simulink model "TADPOLE_Closed_Loop_CTRL2"  (R2024b)
settings: Solver=ode45  StartTime=0.0  StopTime=19  RelTol=1e-3
InitFcn:
  | clear mex;
values from neighbouring files (symbols this model uses):
  timeDelta = 1/5000    (= 0.0002)    [TADPOLEControl.m]
undefined symbols (not defined in the file or in its folder): DiscIntNeverNeededParam
settings Model: PacingRate=2  Creator=pplat  LastModifiedBy=pplat
settings DebuggingCC: AlgebraicLoopMsg=none

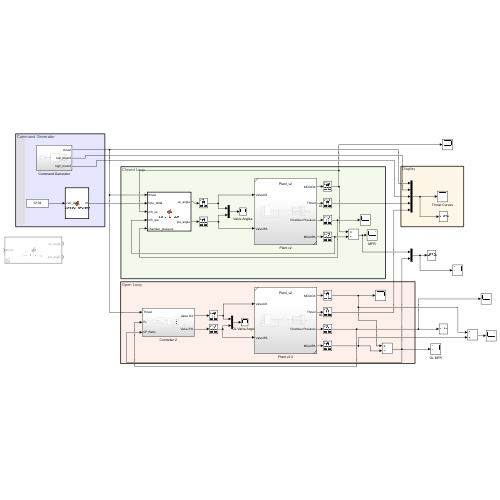
[thumbnail: Simulink's stored preview of the top-level diagram]
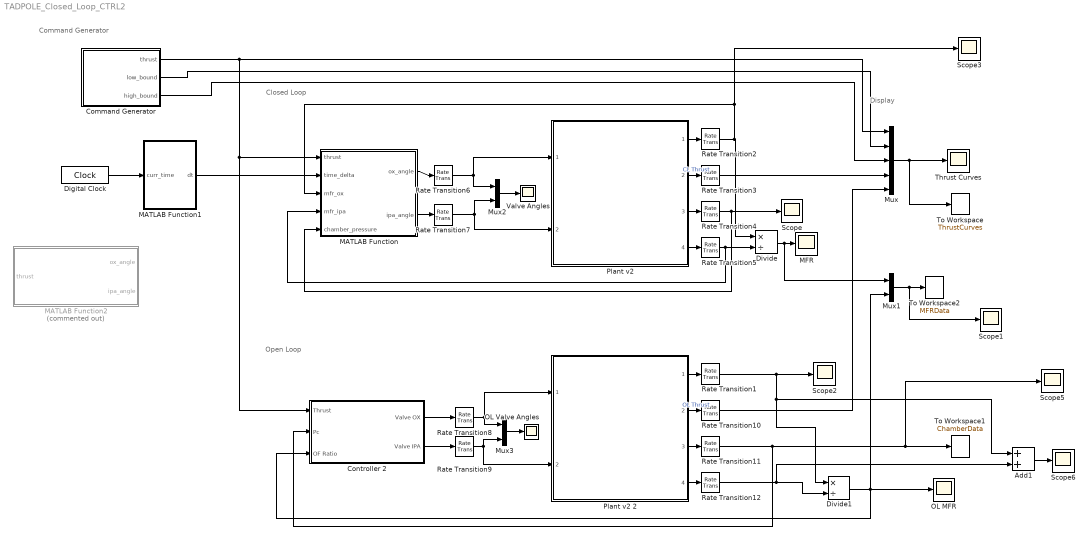
== system TADPOLE_Closed_Loop_CTRL2 ==
  note: Display
  note: Open Loop
  note: Closed Loop
  note: Command Generator
  Add1 : Sum
  Command Generator : Subsystem
  Controller 2 : Subsystem
  Digital Clock : DigitalClock  SampleTime=timeDelta
  Divide : Product  Inputs=*/
  Divide1 : Product  Inputs=*/
  MATLAB Function : MATLAB Function  TreatAsAtomicUnit=on
  MATLAB Function1 : MATLAB Function  TreatAsAtomicUnit=on
  MATLAB Function2 : MATLAB Function  Commented=on  TreatAsAtomicUnit=on
  MFR : Scope
  Mux : Mux  Inputs=5
  Mux1 : Mux  Inputs=2
  Mux2 : Mux  Inputs=2
  Mux3 : Mux  Inputs=2
  OL MFR : Scope
  OL Valve Angles : Scope
  Plant v2 : Subsystem  ReferencedSubsystem=Plant_v2
  Plant v2 2 : Subsystem  ReferencedSubsystem=Plant_v2
  Rate Transition{1..5,10..12} (8 alike) : RateTransition  OutPortSampleTime=timeDeltaOUT
  Rate Transition{6..9} (4 alike) : RateTransition  OutPortSampleTime=timeDeltaCMD
  Scope{,1..3,5..6} (6 alike) : Scope
  Thrust Curves : Scope
  To Workspace : ToWorkspace  VariableName=ThrustCurves  SaveFormat=Timeseries  SampleTime=-1
  To Workspace1 : ToWorkspace  VariableName=ChamberData  SaveFormat=Timeseries  SampleTime=-1
  To Workspace2 : ToWorkspace  VariableName=MFRData  SaveFormat=Timeseries  SampleTime=-1
  Valve Angles : Scope
  wires:
  Mux/1 -> To Workspace/1, Thrust Curves/1
  Plant v2/4 -> Rate Transition5/1
  MATLAB Function/2(ipa_angle) -> Rate Transition7/1
  MATLAB Function/1(ox_angle) -> Rate Transition6/1
  Mux2/1 -> Valve Angles/1
  Divide/1 -> Mux1/1, MFR/1
  Command Generator/1(thrust) -> Mux/1, Controller 2/1(Thrust), MATLAB Function/1(thrust)
  Plant v2/2 -> Rate Transition3/1  "CL Thrust"
  Command Generator/2(low_bound) -> Mux/2
  Command Generator/3(high_bound) -> Mux/3
  MATLAB Function1/1(dt) -> MATLAB Function/2(time_delta)
  Mux3/1 -> OL Valve Angles/1
  Divide1/1 -> Mux1/2, Controller 2/3(OF Ratio), OL MFR/1
  Controller 2/1(Valve OX) -> Rate Transition8/1
  Controller 2/2(Valve IPA) -> Rate Transition9/1
  Digital Clock/1 -> MATLAB Function1/1(curr_time)
  Plant v2 2/1 -> Rate Transition1/1
  Plant v2 2/4 -> Rate Transition12/1
  Mux1/1 -> Scope1/1, To Workspace2/1
  Plant v2/3 -> Rate Transition4/1
  Plant v2 2/3 -> Rate Transition11/1
  Plant v2/1 -> Rate Transition2/1
  Add1/1 -> Scope6/1
  Rate Transition2/1 -> Divide/1, Scope3/1, MATLAB Function/3(mfr_ox)
  Rate Transition3/1 -> Mux/4
  Rate Transition4/1 -> MATLAB Function/5(chamber_pressure), Scope/1
  Rate Transition5/1 -> Divide/2, MATLAB Function/4(mfr_ipa)
  Rate Transition6/1 -> Plant v2/1, Mux2/1
  Rate Transition7/1 -> Plant v2/2, Mux2/2
  Rate Transition8/1 -> Plant v2 2/1, Mux3/1
  Rate Transition9/1 -> Plant v2 2/2, Mux3/2
  Rate Transition1/1 -> Scope2/1, Add1/1, Divide1/1
  Rate Transition10/1 -> Mux/5
  Plant v2 2/2 -> Rate Transition10/1  "OL Thrust"
  Rate Transition11/1 -> Controller 2/2(Pc), Scope5/1, To Workspace1/1
  Rate Transition12/1 -> Add1/2, Divide1/2

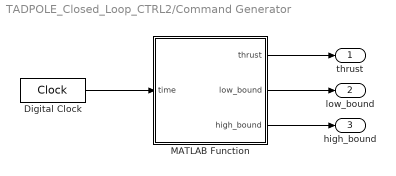
== system TADPOLE_Closed_Loop_CTRL2/Command Generator ==
  Digital Clock : DigitalClock  SampleTime=timeDelta
  MATLAB Function : MATLAB Function  TreatAsAtomicUnit=on
  thrust : Outport
  low_bound : Outport  Port=2
  high_bound : Outport  Port=3
  wires:
  MATLAB Function/1(thrust) -> thrust/1
  Digital Clock/1 -> MATLAB Function/1(time)
  MATLAB Function/2(low_bound) -> low_bound/1
  MATLAB Function/3(high_bound) -> high_bound/1

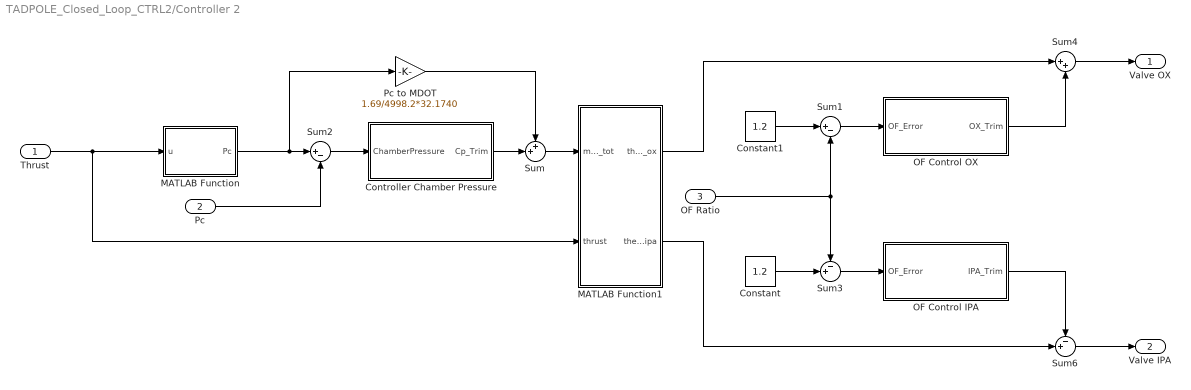
== system TADPOLE_Closed_Loop_CTRL2/Controller 2 ==
  Thrust : Inport
  Pc : Inport  Port=2
  OF Ratio : Inport  Port=3
  Constant : Constant  Value=1.2
  Constant1 : Constant  Value=1.2
  Controller Chamber Pressure : Subsystem
      settings: PortSchema="{\"entries\":[{\"content\":{\"sides\":[{\"content\":{\"connectorIds\":[\"Out1\"]},\"type\":\"ConnectorPlacement.EquallySpacedRectSide\",\"uuid\":\"33f68c87-1ae2-45d4-8ad9-4cf3c5bc8584\"},{\"content\":{\"connectorIds\":[\"In1\"],\"side\":\"RIGHT\"},\"type\":\"ConnectorPlacement.EquallySpacedRectSide\",\"uuid\":\"17976ab6-0faa-4d7d-91ba-f8a21a62dc32\"},{\"content\":{\"side\":\"TOP\"},\"type\":\"ConnectorPlacement.EquallySpacedRectSide\",\"uuid\":\"89a256ba-7dd2-41f4-a68b-27cc674e20da\"},{\"content\":{\"side\":\"BOTTOM\"},\"type\":\"ConnectorPlacement.EquallySpacedRectSide\",\"uuid\":\"73e60893-e40b-4ea1-8c2d-1d944b0843d3\"}]},\"type\":\"ConnectorPlacement.EquallySpacedConnector\",\"uuid\":\"c17bed4f-f3ae-43fd-abcb-ba9ac56db614\"}],\"packageUris\":[\"http://schema.mathworks.com/mf0/Connector/R2020b\"],\"version\":\"1.0\"}"
  MATLAB Function : MATLAB Function  TreatAsAtomicUnit=on
  MATLAB Function1 : MATLAB Function  TreatAsAtomicUnit=on
  OF Control IPA : Subsystem
      settings: PortSchema="{\"entries\":[{\"content\":{\"sides\":[{\"content\":{\"connectorIds\":[\"Out1\"]},\"type\":\"ConnectorPlacement.EquallySpacedRectSide\",\"uuid\":\"33f68c87-1ae2-45d4-8ad9-4cf3c5bc8584\"},{\"content\":{\"connectorIds\":[\"In1\"],\"side\":\"RIGHT\"},\"type\":\"ConnectorPlacement.EquallySpacedRectSide\",\"uuid\":\"17976ab6-0faa-4d7d-91ba-f8a21a62dc32\"},{\"content\":{\"side\":\"TOP\"},\"type\":\"ConnectorPlacement.EquallySpacedRectSide\",\"uuid\":\"89a256ba-7dd2-41f4-a68b-27cc674e20da\"},{\"content\":{\"side\":\"BOTTOM\"},\"type\":\"ConnectorPlacement.EquallySpacedRectSide\",\"uuid\":\"73e60893-e40b-4ea1-8c2d-1d944b0843d3\"}]},\"type\":\"ConnectorPlacement.EquallySpacedConnector\",\"uuid\":\"c17bed4f-f3ae-43fd-abcb-ba9ac56db614\"}],\"packageUris\":[\"http://schema.mathworks.com/mf0/Connector/R2020b\"],\"version\":\"1.0\"}"
  OF Control OX : Subsystem
      settings: PortSchema="{\"entries\":[{\"content\":{\"sides\":[{\"content\":{\"connectorIds\":[\"Out1\"]},\"type\":\"ConnectorPlacement.EquallySpacedRectSide\",\"uuid\":\"33f68c87-1ae2-45d4-8ad9-4cf3c5bc8584\"},{\"content\":{\"connectorIds\":[\"In1\"],\"side\":\"RIGHT\"},\"type\":\"ConnectorPlacement.EquallySpacedRectSide\",\"uuid\":\"17976ab6-0faa-4d7d-91ba-f8a21a62dc32\"},{\"content\":{\"side\":\"TOP\"},\"type\":\"ConnectorPlacement.EquallySpacedRectSide\",\"uuid\":\"89a256ba-7dd2-41f4-a68b-27cc674e20da\"},{\"content\":{\"side\":\"BOTTOM\"},\"type\":\"ConnectorPlacement.EquallySpacedRectSide\",\"uuid\":\"73e60893-e40b-4ea1-8c2d-1d944b0843d3\"}]},\"type\":\"ConnectorPlacement.EquallySpacedConnector\",\"uuid\":\"c17bed4f-f3ae-43fd-abcb-ba9ac56db614\"}],\"packageUris\":[\"http://schema.mathworks.com/mf0/Connector/R2020b\"],\"version\":\"1.0\"}"
  Pc to MDOT : Gain  Gain=1.69/4998.2*32.1740
  Sum : Sum  Inputs=++|
  Sum1 : Sum  Inputs=|+-
  Sum2 : Sum  Inputs=|+-
  Sum3 : Sum  Inputs=-+|
  Sum4 : Sum  Inputs=|++
  Sum6 : Sum  Inputs=-+|
  Valve OX : Outport
  Valve IPA : Outport  Port=2
  wires:
  Thrust/1 -> MATLAB Function1/2(thrust), MATLAB Function/1(u)
  MATLAB Function/1(Pc) -> Sum2/1, Pc to MDOT/1
  Sum/1 -> MATLAB Function1/1(mdot_tot)
  Pc to MDOT/1 -> Sum/1
  Pc/1 -> Sum2/2
  Sum2/1 -> Controller Chamber Pressure/1(ChamberPressure)
  Controller Chamber Pressure/1(Cp_Trim) -> Sum/2
  Constant1/1 -> Sum1/1
  OF Ratio/1 -> Sum3/1, Sum1/2
  Constant/1 -> Sum3/2
  Sum3/1 -> OF Control IPA/1(OF_Error)
  Sum1/1 -> OF Control OX/1(OF_Error)
  MATLAB Function1/1(theta_ox) -> Sum4/1
  Sum4/1 -> Valve OX/1
  MATLAB Function1/2(theta_ipa) -> Sum6/2
  Sum6/1 -> Valve IPA/1
  OF Control IPA/1(IPA_Trim) -> Sum6/1
  OF Control OX/1(OX_Trim) -> Sum4/2

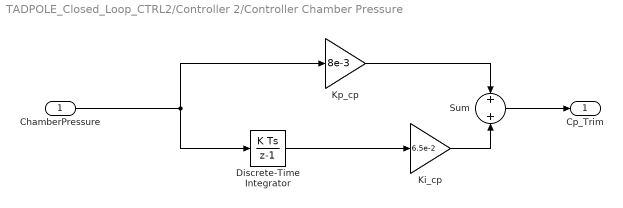
== system TADPOLE_Closed_Loop_CTRL2/Controller 2/Controller Chamber Pressure ==
  ChamberPressure : Inport
  Discrete-Time Integrator : DiscreteIntegrator  SampleTime=-1  ICPrevOutput=DiscIntNeverNeededParam  ICPrevScaledInput=DiscIntNeverNeededParam
  Ki_cp : Gain  Gain=6.5e-2
  Kp_cp : Gain  Gain=8e-3
  Sum : Sum  Inputs=+|+
  Cp_Trim : Outport
  wires:
  Kp_cp/1 -> Sum/1
  Ki_cp/1 -> Sum/2
  Sum/1 -> Cp_Trim/1
  Discrete-Time Integrator/1 -> Ki_cp/1
  ChamberPressure/1 -> Discrete-Time Integrator/1, Kp_cp/1

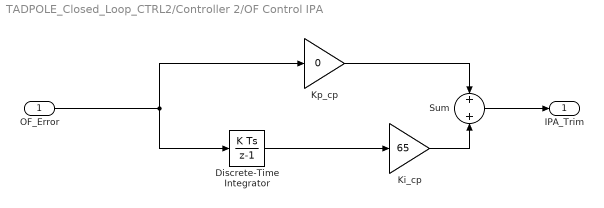
== system TADPOLE_Closed_Loop_CTRL2/Controller 2/OF Control IPA ==
  OF_Error : Inport
  Discrete-Time Integrator : DiscreteIntegrator  SampleTime=-1  ICPrevOutput=DiscIntNeverNeededParam  ICPrevScaledInput=DiscIntNeverNeededParam
  Ki_cp : Gain  Gain=65
  Kp_cp : Gain  Gain=0
  Sum : Sum  Inputs=+|+
  IPA_Trim : Outport
  wires:
  OF_Error/1 -> Kp_cp/1, Discrete-Time Integrator/1
  Discrete-Time Integrator/1 -> Ki_cp/1
  Sum/1 -> IPA_Trim/1
  Ki_cp/1 -> Sum/2
  Kp_cp/1 -> Sum/1

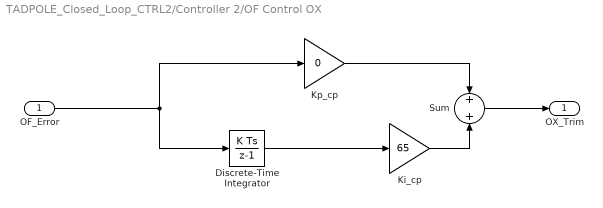
== system TADPOLE_Closed_Loop_CTRL2/Controller 2/OF Control OX ==
  OF_Error : Inport
  Discrete-Time Integrator : DiscreteIntegrator  SampleTime=-1  ICPrevOutput=DiscIntNeverNeededParam  ICPrevScaledInput=DiscIntNeverNeededParam
  Ki_cp : Gain  Gain=65
  Kp_cp : Gain  Gain=0
  Sum : Sum  Inputs=+|+
  OX_Trim : Outport
  wires:
  OF_Error/1 -> Kp_cp/1, Discrete-Time Integrator/1
  Discrete-Time Integrator/1 -> Ki_cp/1
  Sum/1 -> OX_Trim/1
  Ki_cp/1 -> Sum/2
  Kp_cp/1 -> Sum/1

== matlab function TADPOLE_Closed_Loop_CTRL2/MATLAB Function ==
  data: thrust input; time_delta input; ox_angle output; ipa_angle output; mfr_ox input; mfr_ipa input; chamber_pressure input
function [ox_angle, ipa_angle] = send_to_cpp(thrust, time_delta, mfr_ox, mfr_ipa, chamber_pressure)
coder.extrinsic('closed_loop_valve_control_wrap');  % Declare MEX function as extrinsic
ox_angle = 0;
ipa_angle = 0;
[ox_angle, ipa_angle] = closed_loop_valve_control_wrap(thrust, time_delta, mfr_ox, mfr_ipa, chamber_pressure);

== matlab function TADPOLE_Closed_Loop_CTRL2/MATLAB Function1 ==
  data: dt output; curr_time input
function dt = measure_timestep(curr_time)
    persistent prev_time;
    if isempty(prev_time)
        prev_time = 0;
    end
    if curr_time < 0.3
        dt = 0;
    else
        dt = curr_time - prev_time;
    end
    prev_time = curr_time;
end

== matlab function TADPOLE_Closed_Loop_CTRL2/Command Generator/MATLAB Function ==
  data: time input; thrust output; low_bound output; high_bound output
function [thrust,low_bound,high_bound] = thrustCurveBounds(time)
thrust = test4(time);
t_past = test4(time - 0.5);
t_future = test4(time + 0.5);

high_bound = max([thrust, t_past, t_future]) + 0.05 * 550;
low_bound = min([thrust, t_past, t_future]) - 0.05 * 550;

end

== matlab function TADPOLE_Closed_Loop_CTRL2/MATLAB Function2 ==
  data: thrust input; ox_angle output; ipa_angle output
function [ox_angle, ipa_angle] = send_to_cpp(thrust)
coder.extrinsic('open_loop_valve_control_wrap');  % Declare MEX function as extrinsic
ox_angle = 0;
ipa_angle = 0;
[ox_angle, ipa_angle] = open_loop_valve_control_wrap(thrust);

== matlab function TADPOLE_Closed_Loop_CTRL2/Controller 2/MATLAB Function ==
  data: u input; Pc output
function Pc = T2PC(u)

    Pc = thrust_to_cp(u);
end

== matlab function TADPOLE_Closed_Loop_CTRL2/Controller 2/MATLAB Function1 ==
  data: mdot_tot input; theta_ox output; thrust input; theta_ipa output
function [theta_ox, theta_ipa] = angles(mdot_tot, thrust)

    [theta_ox, theta_ipa] = mdot2valves(mdot_tot, thrust);
end
